simulink model "sim_with_sensors_sim"  (R2023b)
settings: Solver=ode5  StartTime=0.0  StopTime=1000  FixedStep=Auto  RelTol=1e-3
values from neighbouring files (symbols this model uses):
  a = R_E+500*1e3    (= 6871000)    [Sensors.m]    (also in sim_with_sensors.m = 6851.22197053; simulation_with_sensors.m = 26584)
  A0 = eye(3)    [sim_with_sensors.m]
  e = 0    [Sensors.m]    (also in sim_with_sensors.m = 0.00183012221618; simulation_with_sensors.m = 0.00023103)
  H0 = sqrt(g01^2+g11^2+h11^2)*1e-9    [sim_with_sensors.m]    (also in simulation_with_sensors.m)
  I = diag([I1 I2 I3])*1e-9    [sim_with_sensors.m]    (also in simulation_with_sensors.m = diag([100.09 25.1 91.6]))
  Iinv = I\eye(3)    [sim_with_sensors.m]
  incl = deg2rad(11.5)    [sim_with_sensors.m]    (also in simulation_with_sensors.m)
  jb = [0.01; 0.05; 0.01]    [sim_with_sensors.m]
  k_gain = (4*pi/T) * (1 + sin(chsi)) * I1 *1e-9    [sim_with_sensors.m]
  mu = astroConstants(13)    [sim_with_sensors.m]
  n = n+1    (= 1)    [Sensors.m]    (also in sim_with_sensors.m = sqrt(mu/a^3); simulation_with_sensors.m = sqrt(astroConstants(13) / a^3))
  omega0 = [0.01; 0.01; 0.01]*6    [sim_with_sensors.m]
  omegaE = deg2rad(15)/3600    [sim_with_sensors.m]    (also in simulation_with_sensors.m)
  R_mat = om_matrix * i_matrix * OM_matrix    [sim_with_sensors.m]
  Rt = astroConstants(23)    [sim_with_sensors.m]
  s0 = zeros(3,1)    [sim_with_sensors.m]    (also in simulation_with_sensors.m = [0; 0; 0])
  theta0 = 3.109851878856139    (= 3.10985187886)    [sim_with_sensors.m]
undefined symbols (not defined in the file or in its folder): phi0, psi0
libraries: matrix_library x11, simulink x7, dspmathops x6, vrlib x3, dspfdesign x1
settings Model: Creator=marcellopareschi  LastModifiedBy=danie

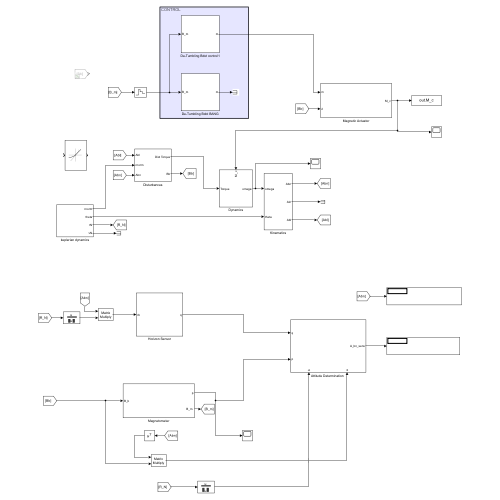
[thumbnail: Simulink's stored preview of the top-level diagram]
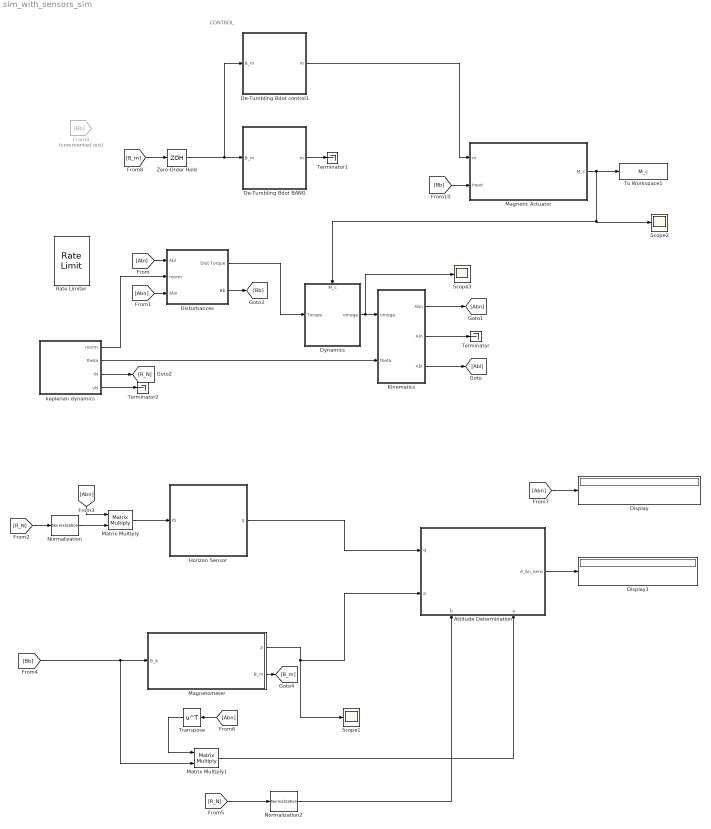
== system sim_with_sensors_sim ==
  note: CONTROL
  "Attitude Determination  " : Subsystem
      settings: PortSchema="{\"entries\":[{\"content\":{\"sides\":[{\"content\":{\"connectorIds\":[\"In1\",\"In2\"]},\"type\":\"ConnectorPlacement.EquallySpacedRectSide\",\"uuid\":\"730966cf-d0d7-44a0-92f0-b5324480e7cc\"},{\"content\":{\"connectorIds\":[\"Out1\"],\"side\":\"RIGHT\"},\"type\":\"ConnectorPlacement.EquallySpacedRectSide\",\"uuid\":\"c83e6b57-46fe-4a45-9824-d3495e15bf6a\"},{\"content\":{\"side\":\"TOP\"},\"type\":\"ConnectorPlacement.EquallySpacedRectSide\",\"uuid\":\"4938c298-c2b3-45b7-bcb0-70b8132dabc6\"},{\"content\":{\"connectorIds\":[\"In3\",\"In4\"],\"side\":\"BOTTOM\"},\"type\":\"ConnectorPlacement.EquallySpacedRectSide\",\"uuid\":\"6d6a244e-80db-423b-a0a5-9a5face48fcb\"}]},\"type\":\"ConnectorPlacement.EquallySpacedConnector\",\"uuid\":\"7eb6767d-3ff0-4577-86c9-ebc5e763f220\"}],\"packageUris\":[\"http://schema.mathworks.com/mf0/Connector/R2020b\"],\"version\":\"1.0\"}"
  De-Tumbling Bdot BANG : Subsystem
  De-Tumbling Bdot control1 : Subsystem
  Display : Display
  Display1 : Display
  Disturbances : Subsystem
  Dynamics : Subsystem
      settings: PortSchema="{\"entries\":[{\"content\":{\"sides\":[{\"content\":{\"connectorIds\":[\"In1\"]},\"type\":\"ConnectorPlacement.EquallySpacedRectSide\",\"uuid\":\"c50eaaef-bc5a-4b30-975a-dad3b72c53e1\"},{\"content\":{\"connectorIds\":[\"Out1\"],\"side\":\"RIGHT\"},\"type\":\"ConnectorPlacement.EquallySpacedRectSide\",\"uuid\":\"08d23e91-5daf-4f03-95f9-71d6696597c3\"},{\"content\":{\"connectorIds\":[\"In2\"],\"side\":\"TOP\"},\"type\":\"ConnectorPlacement.EquallySpacedRectSide\",\"uuid\":\"7ec65280-cc3e-44b1-8843-81c3a216d755\"}]},\"type\":\"ConnectorPlacement.EquallySpacedConnector\",\"uuid\":\"721d018a-ab6c-4a15-8dbf-409a72b03ba1\"}],\"packageUris\":[\"http://schema.mathworks.com/mf0/Connector/R2020b\"],\"version\":\"1.0\"}"
  From9 : From  Commented=on  GotoTag=Bb
  Horizon Sensor : Subsystem
  Kinematics : Subsystem
  Magnetic Actuator : Subsystem
  Magnetometer : Subsystem
  Matrix Multiply : Product  Multiplication=Matrix(*)
  Matrix Multiply1 : Product  Multiplication=Matrix(*)
  Normalization : dspmathops/Normalization  NormType=2-norm  Bias=1e-10  NormOver=Each column  Dimension=1  roundingMode=Floor  overflowMode=off  accumDataTypeStr=Inherit: Same as product output  accumLastDataTypeStr=Inherit: Same as product output  outputDataTypeStr=Inherit: Same as product output  outputMin=[]  outputMax=[]  outputLastDataTypeStr=Inherit: Same as product output
  Normalization2 : dspmathops/Normalization  NormType=2-norm  Bias=1e-10  NormOver=Each column  Dimension=1  roundingMode=Floor  overflowMode=off  accumDataTypeStr=Inherit: Same as product output  accumLastDataTypeStr=Inherit: Same as product output  outputDataTypeStr=Inherit: Same as product output  outputMin=[]  outputMax=[]  outputLastDataTypeStr=Inherit: Same as product output
  Rate Limiter : RateLimiter  SampleTimeMode=inherited
  Scope1 : Scope
  Scope2 : Scope
  Scope3 : Scope
  Terminator : Terminator
  Terminator1 : Terminator
  Terminator2 : Terminator
  To Workspace1 : ToWorkspace  VariableName=M_c  SampleTime=-1
  Transpose : Math  Operator=transpose
  Zero-Order Hold : ZeroOrderHold  SampleTime=1/30
  keplerian dynamics : Subsystem
  wires:
  Dynamics/1(omega) -> Scope3/1, Kinematics/1(omega)
  keplerian dynamics/2(theta) -> Kinematics/2(theta)
  keplerian dynamics/1(rnorm) -> Disturbances/2(rnorm)
  Disturbances/1(Dist Torque) -> Dynamics/1(Torque)
  Kinematics/2(Aln) -> Terminator/1
  Kinematics/3(Abl) -> [Abl]
  [Abl] -> Disturbances/1(Abl)
  Kinematics/1(Abn) -> [Abn]
  [Abn] -> Disturbances/3(Abn)
  keplerian dynamics/4(vN) -> Terminator2/1
  keplerian dynamics/3(rN) -> [R_N]
  [R_N] -> Normalization/1
  Normalization/1 -> Matrix Multiply/2
  [Abn] -> Matrix Multiply/1
  Matrix Multiply/1 -> Horizon Sensor/1(rb)
  Disturbances/2(Bb) -> [Bb]
  [Bb] -> Matrix Multiply1/2, Magnetometer/1(B_b)
  [R_N] -> Normalization2/1
  [Abn] -> Transpose/1
  Transpose/1 -> Matrix Multiply1/1
  Horizon Sensor/1(q) -> "Attitude Determination  "/1(q)
  Magnetometer/1(p) -> Scope1/1, "Attitude Determination  "/2(p)
  Normalization2/1 -> "Attitude Determination  "/3(b)
  Matrix Multiply1/1 -> "Attitude Determination  "/4(a)
  [Abn] -> Display/1
  "Attitude Determination  "/1(A_bn_sens) -> Display1/1
  De-Tumbling Bdot control1/1(m) -> Magnetic Actuator/1(m)
  Magnetometer/2("B_m ") -> [B_m]
  Zero-Order Hold/1 -> De-Tumbling Bdot control1/1(B_m), De-Tumbling Bdot BANG/1(B_m)
  [B_m] -> Zero-Order Hold/1
  [Bb] -> Magnetic Actuator/2(Input)
  De-Tumbling Bdot BANG/1(m) -> Terminator1/1
  Magnetic Actuator/1(M_c) -> Scope2/1, Dynamics/2(M_c), To Workspace1/1

== system sim_with_sensors_sim/Attitude Determination   ==
  q : Inport
  p : Inport  Port=2
  b : Inport  Port=3
  a : Inport  Port=4
  Matrix Multiply : Product  Multiplication=Matrix(*)
  S : Subsystem
  Transpose : Math  Operator=transpose
  V : Subsystem
  A_bn_sens : Outport
  wires:
  q/1 -> S/1(q)
  p/1 -> S/2(p)
  a/1 -> V/2(a)
  b/1 -> V/1(b)
  V/1(V) -> Transpose/1
  S/1(S) -> Matrix Multiply/1
  Transpose/1 -> Matrix Multiply/2
  Matrix Multiply/1 -> A_bn_sens/1

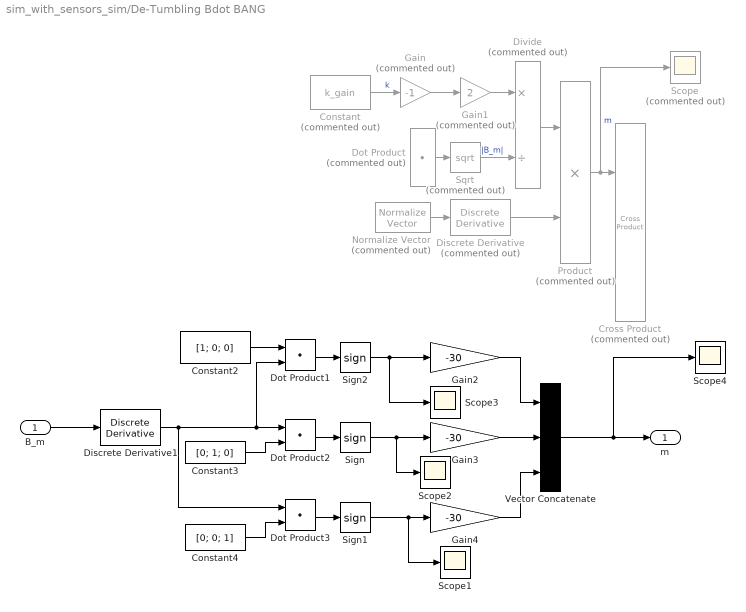
== system sim_with_sensors_sim/De-Tumbling Bdot BANG ==
  B_m : Inport
  Constant : Constant  Commented=on  Value=k_gain
  Constant2 : Constant  Value=[1; 0; 0]  SampleTime=1/30
  Constant3 : Constant  Value=[0; 1; 0]  SampleTime=1/30
  Constant4 : Constant  Value=[0; 0; 1]  SampleTime=1/30
  Cross Product : matrix_library/Cross Product  Commented=on
  Discrete Derivative : simulink/Discrete/Discrete Derivative  Commented=on  gainval=1.0  ICPrevScaledInput=0.0  OutMin=[]  OutMax=[]  OutDataType=fixdt(1, 16)  OutScaling=2^-10  DoSatur=off
  Discrete Derivative1 : simulink/Discrete/Discrete Derivative  gainval=1.0  ICPrevScaledInput=0.0  OutMin=[]  OutMax=[]  OutDataType=fixdt(1, 16)  OutScaling=2^-10  DoSatur=off
  Divide : Product  Commented=on  Inputs=*/
  Dot Product : DotProduct  Commented=on  OutDataTypeStr=Inherit: Inherit via internal rule
  Dot Product1 : DotProduct  OutDataTypeStr=Inherit: Inherit via internal rule
  Dot Product2 : DotProduct  OutDataTypeStr=Inherit: Inherit via internal rule
  Dot Product3 : DotProduct  OutDataTypeStr=Inherit: Inherit via internal rule
  Gain : Gain  Commented=on  Gain=-1
  Gain1 : Gain  Commented=on  Gain=2
  Gain2 : Gain  Gain=-30
  Gain3 : Gain  Gain=-30
  Gain4 : Gain  Gain=-30
  Normalize Vector : vrlib/Utilities/Normalize Vector  Commented=on  maxzero=0
  Product : Product  Commented=on
  Scope : Scope  Commented=on
  Scope{1..4} (4 alike) : Scope
  Sign : Signum
  Sign1 : Signum
  Sign2 : Signum
  Sqrt : Sqrt  Commented=on
  Vector Concatenate : Concatenate  NumInputs=3
  m : Outport
  wires:
  Gain1/1 -> Divide/1
  Normalize Vector/1 -> Discrete Derivative/1
  Sqrt/1 -> Divide/2  "|B_m|"
  Product/1 -> Cross Product/1, Scope/1  "m"
  Discrete Derivative/1 -> Product/2
  Divide/1 -> Product/1
  Gain/1 -> Gain1/1
  Constant/1 -> Gain/1  "k"
  Dot Product/1 -> Sqrt/1
  Discrete Derivative1/1 -> Dot Product3/1, Dot Product2/1, Dot Product1/2
  B_m/1 -> Discrete Derivative1/1
  Constant2/1 -> Dot Product1/1
  Constant3/1 -> Dot Product2/2
  Constant4/1 -> Dot Product3/2
  Dot Product3/1 -> Sign1/1
  Dot Product2/1 -> Sign/1
  Dot Product1/1 -> Sign2/1
  Sign2/1 -> Scope3/1, Gain2/1
  Sign/1 -> Scope2/1, Gain3/1
  Sign1/1 -> Scope1/1, Gain4/1
  Gain3/1 -> Vector Concatenate/2
  Gain4/1 -> Vector Concatenate/3
  Gain2/1 -> Vector Concatenate/1
  Vector Concatenate/1 -> m/1, Scope4/1

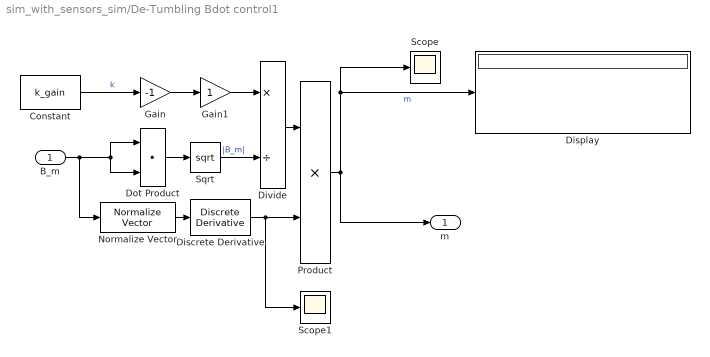
== system sim_with_sensors_sim/De-Tumbling Bdot control1 ==
  B_m : Inport
  Constant : Constant  Value=k_gain
  Discrete Derivative : simulink/Discrete/Discrete Derivative  gainval=1.0  ICPrevScaledInput=0.0  OutMin=[]  OutMax=[]  OutDataType=fixdt(1, 16)  OutScaling=2^-10  DoSatur=off
  Display : Display
  Divide : Product  Inputs=*/
  Dot Product : DotProduct  OutDataTypeStr=Inherit: Inherit via internal rule
  Gain : Gain  Gain=-1
  Gain1 : Gain
  Normalize Vector : vrlib/Utilities/Normalize Vector  maxzero=0
  Product : Product
  Scope : Scope
  Scope1 : Scope
  Sqrt : Sqrt
  m : Outport
  wires:
  Dot Product/1 -> Sqrt/1
  Constant/1 -> Gain/1  "k"
  Gain/1 -> Gain1/1
  Divide/1 -> Product/1
  Discrete Derivative/1 -> Scope1/1, Product/2
  Product/1 -> m/1, Scope/1, Display/1  "m"
  Sqrt/1 -> Divide/2  "|B_m|"
  Gain1/1 -> Divide/1
  Normalize Vector/1 -> Discrete Derivative/1
  B_m/1 -> Normalize Vector/1, Dot Product/2, Dot Product/1

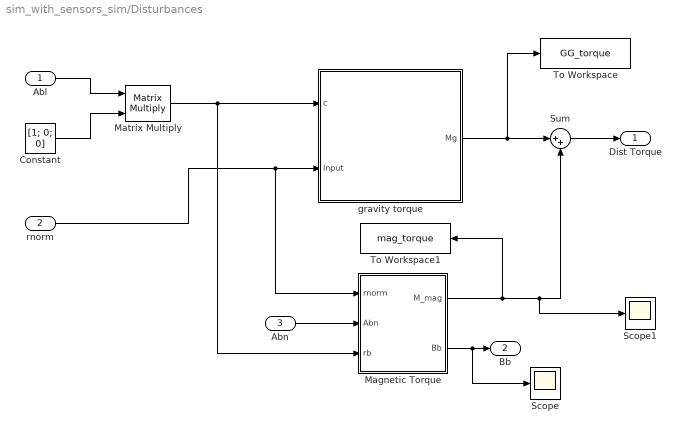
== system sim_with_sensors_sim/Disturbances ==
  Abl : Inport
  rnorm : Inport  Port=2
  Abn : Inport  Port=3
  Constant : Constant  Value=[1; 0; 0]
  "Magnetic Torque " : Subsystem
  Matrix Multiply : Product  Multiplication=Matrix(*)
  Scope : Scope
  Scope1 : Scope
  Sum : Sum  Inputs=|++
  To Workspace : ToWorkspace  VariableName=GG_torque  SampleTime=-1
  To Workspace1 : ToWorkspace  VariableName=mag_torque  SampleTime=-1
  gravity torque : Subsystem
  Dist Torque : Outport
  Bb : Outport  Port=2
  wires:
  Abl/1 -> Matrix Multiply/1
  Constant/1 -> Matrix Multiply/2
  Matrix Multiply/1 -> "Magnetic Torque "/3(rb), gravity torque/1(c)
  rnorm/1 -> "Magnetic Torque "/1(rnorm), gravity torque/2(Input)
  Abn/1 -> "Magnetic Torque "/2(Abn)
  gravity torque/1(Mg) -> To Workspace/1, Sum/1
  "Magnetic Torque "/1(M_mag) -> To Workspace1/1, Scope1/1, Sum/2
  Sum/1 -> Dist Torque/1
  "Magnetic Torque "/2(Bb) -> Scope/1, Bb/1

== system sim_with_sensors_sim/Dynamics ==
  Torque : Inport
  M_c : Inport  Port=2
  Constant : Constant  Value=I
  Constant1 : Constant  Value=Iinv
  Cross Product : matrix_library/Cross Product
  Integrator : Integrator  InitialCondition=omega0
  Product : Product  Multiplication=Matrix(*)
  Product1 : Product  Multiplication=Matrix(*)
  Scope : Scope
  Scope1 : Scope
  Sum : Sum  Inputs=+++
  To Workspace : ToWorkspace  VariableName=omegab  SampleTime=-1
  omega : Outport
  wires:
  Constant/1 -> Product/1
  Product1/1 -> Integrator/1
  Integrator/1 -> omega/1, To Workspace/1, Scope/1, Product/2, Cross Product/2
  Product/1 -> Cross Product/1
  Constant1/1 -> Product1/1
  Cross Product/1 -> Sum/2
  Sum/1 -> Product1/2
  Torque/1 -> Sum/3
  M_c/1 -> Scope1/1, Sum/1

== system sim_with_sensors_sim/Horizon Sensor ==
  rb : Inport
  Cross Product : matrix_library/Cross Product
  Normalization1 : dspmathops/Normalization  NormType=2-norm  Bias=1e-10  NormOver=Each column  Dimension=1  roundingMode=Floor  overflowMode=off  accumDataTypeStr=Inherit: Same as product output  accumLastDataTypeStr=Inherit: Same as product output  outputDataTypeStr=Inherit: Same as product output  outputMin=[]  outputMax=[]  outputLastDataTypeStr=Inherit: Same as product output
  Product : Product
  Sum2 : Sum
  Uniform Random Number : UniformRandomNumber  SampleTime=1/30
  Uniform Random Number1 : UniformRandomNumber  SampleTime=1/30
  Uniform Random Number2 : UniformRandomNumber  SampleTime=1/30
  Uniform Random Number3 : UniformRandomNumber  Minimum=0  Maximum=tan(deg2rad(0.1))  SampleTime=1/30
  Vector Concatenate : Concatenate  NumInputs=3
  Zero-Order Hold : ZeroOrderHold  SampleTime=1/30
  q : Outport
  wires:
  Uniform Random Number/1 -> Vector Concatenate/1
  Product/1 -> Sum2/1
  Uniform Random Number1/1 -> Vector Concatenate/2
  Zero-Order Hold/1 -> Cross Product/2, Sum2/2  "R_B"
  Normalization1/1 -> Product/2
  Vector Concatenate/1 -> Cross Product/1
  Uniform Random Number3/1 -> Product/1
  Cross Product/1 -> Normalization1/1
  Uniform Random Number2/1 -> Vector Concatenate/3
  rb/1 -> Zero-Order Hold/1
  Sum2/1 -> q/1  "q"

== system sim_with_sensors_sim/Kinematics ==
  omega : Inport
  theta : Inport  Port=2
  Product : Product  Multiplication=Matrix(*)
  Subsystem1 : Subsystem
  To Workspace : ToWorkspace  VariableName=angles  SampleTime=-1
  Transpose : Math  Operator=transpose
  compute Aln : Subsystem
  Abn : Outport
  Aln : Outport  Port=2
  Abl : Outport  Port=3
  wires:
  omega/1 -> Subsystem1/1(In1)
  Subsystem1/1(Angles) -> To Workspace/1, Subsystem1/2(Input)
  Subsystem1/2(A) -> Product/1, Abn/1, Subsystem1/3(Input1)
  theta/1 -> compute Aln/1(theta)
  compute Aln/1(A_ln) -> Transpose/1, Aln/1
  Transpose/1 -> Product/2
  Product/1 -> Abl/1

== system sim_with_sensors_sim/Magnetic Actuator ==
  m : Inport
  Input : Inport  Port=2
  Band-Limited White Noise : simulink/Sources/Band-Limited White Noise  Cov=[0.1]  Ts=0.1  seed=[23341]
  Cross Product : matrix_library/Cross Product
  Lowpass Filter : dspfdesign/Lowpass Filter  FilterType=FIR  DesignForMinimumOrder=on  FilterOrder=50  PassbandFrequency=100  StopbandFrequency=120  PassbandRipple=0.1  StopbandAttenuation=80  SampleRateMode=Specify on dialog  SampleRate=44100  SimulateUsing=Interpreted execution  roundingMode=Floor  coeffsDataTypeStr=fixdt(1,16)
  Rate Limiter1 : RateLimiter  RisingSlewLimit=10  FallingSlewLimit=-10  SampleTimeMode=inherited
  Saturation : Saturate  UpperLimit=100  LowerLimit=-100
  Scope1 : Scope
  Sum1 : Sum  Inputs=++|
  M_c : Outport
  wires:
  Input/1 -> Cross Product/2  "B_body"
  Cross Product/1 -> M_c/1
  Rate Limiter1/1 -> Saturation/1
  Band-Limited White Noise/1 -> Sum1/1
  m/1 -> Sum1/2
  Sum1/1 -> Rate Limiter1/1
  Saturation/1 -> Lowpass Filter/1
  Lowpass Filter/1 -> Cross Product/1

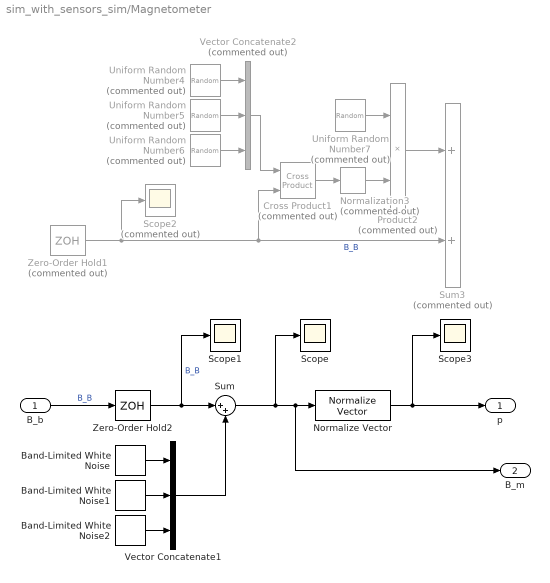
== system sim_with_sensors_sim/Magnetometer ==
  B_b : Inport
  Band-Limited White Noise : simulink/Sources/Band-Limited White Noise  Cov=[1.18^2 *1e-18]  Ts=1/30  seed=[23341]
  Band-Limited White Noise1 : simulink/Sources/Band-Limited White Noise  Cov=[1.18^2 *1e-18]  Ts=1/30  seed=[23341]
  Band-Limited White Noise2 : simulink/Sources/Band-Limited White Noise  Cov=[1.18^2 *1e-18]  Ts=1/30  seed=[23341]
  Cross Product1 : matrix_library/Cross Product  Commented=on
  Normalization3 : dspmathops/Normalization  Commented=on  NormType=2-norm  Bias=1e-10  NormOver=Each column  Dimension=1  roundingMode=Floor  overflowMode=off  accumDataTypeStr=Inherit: Same as product output  accumLastDataTypeStr=Inherit: Same as product output  outputDataTypeStr=Inherit: Same as product output  outputMin=[]  outputMax=[]  outputLastDataTypeStr=Inherit: Same as product output
  Normalize Vector : vrlib/Utilities/Normalize Vector  maxzero=0
  Product2 : Product  Commented=on
  Scope : Scope
  Scope1 : Scope
  Scope2 : Scope  Commented=on
  Scope3 : Scope
  Sum : Sum  Inputs=|++
  Sum3 : Sum  Commented=on
  Uniform Random Number4 : UniformRandomNumber  Commented=on  SampleTime=1/30
  Uniform Random Number5 : UniformRandomNumber  Commented=on  SampleTime=1/30
  Uniform Random Number6 : UniformRandomNumber  Commented=on  SampleTime=1/30
  Uniform Random Number7 : UniformRandomNumber  Commented=on  Minimum=0  Maximum=tan(deg2rad(0.5))  SampleTime=1/30
  Vector Concatenate1 : Concatenate  NumInputs=3
  Vector Concatenate2 : Concatenate  Commented=on  NumInputs=3
  Zero-Order Hold1 : ZeroOrderHold  Commented=on  SampleTime=1/30
  Zero-Order Hold2 : ZeroOrderHold  SampleTime=1/30
  p : Outport
  "B_m " : Outport  Port=2
  wires:
  Zero-Order Hold1/1 -> Cross Product1/2, Sum3/2, Scope2/1  "B_B"
  Product2/1 -> Sum3/1
  Normalization3/1 -> Product2/2
  Uniform Random Number4/1 -> Vector Concatenate2/1
  Uniform Random Number6/1 -> Vector Concatenate2/3
  Vector Concatenate2/1 -> Cross Product1/1
  Cross Product1/1 -> Normalization3/1
  Uniform Random Number5/1 -> Vector Concatenate2/2
  Uniform Random Number7/1 -> Product2/1
  B_b/1 -> Zero-Order Hold2/1  "B_B"
  Zero-Order Hold2/1 -> Scope1/1, Sum/1  "B_B"
  Band-Limited White Noise2/1 -> Vector Concatenate1/3
  Band-Limited White Noise1/1 -> Vector Concatenate1/2
  Band-Limited White Noise/1 -> Vector Concatenate1/1
  Normalize Vector/1 -> Scope3/1, p/1
  Vector Concatenate1/1 -> Sum/2
  Sum/1 -> Scope/1, "B_m "/1, Normalize Vector/1

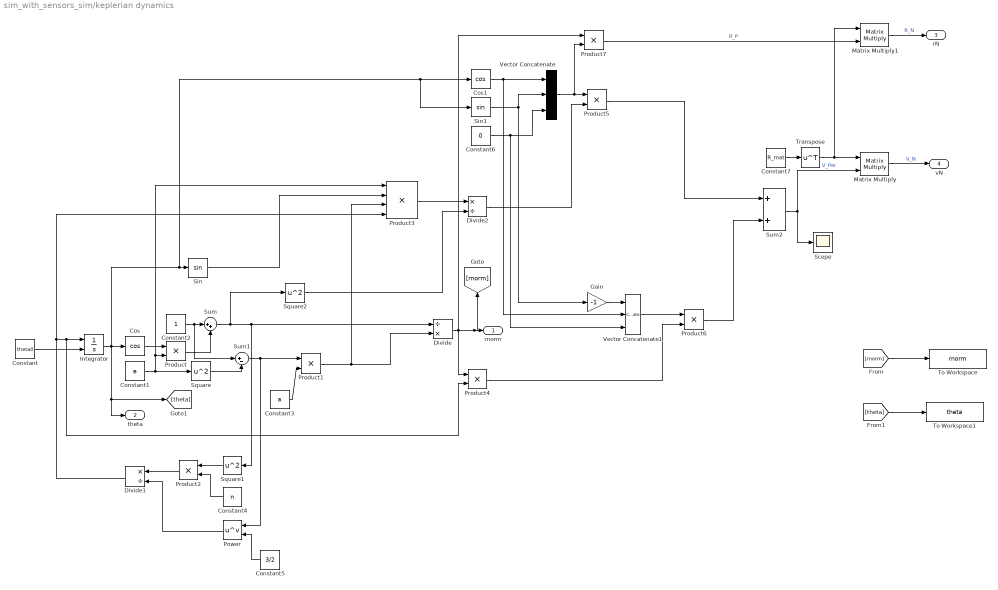
== system sim_with_sensors_sim/keplerian dynamics ==
  Constant : Constant  Value=theta0
  Constant1 : Constant  Value=e
  Constant2 : Constant
  Constant3 : Constant  Value=a
  Constant4 : Constant  Value=n
  Constant5 : Constant  Value=3/2
  Constant6 : Constant  Value=0
  Constant7 : Constant  Value=R_mat
  Cos : Trigonometry  Operator=cos
  Cos1 : Trigonometry  Operator=cos
  Divide : Product  Inputs=/*
  Divide1 : Product  Inputs=*/
  Divide2 : Product  Inputs=*/
  Gain : Gain  Gain=-1
  Integrator : Integrator  InitialConditionSource=external
  Matrix Multiply : Product  Multiplication=Matrix(*)
  Matrix Multiply1 : Product  Multiplication=Matrix(*)
  Power : Math  Operator=pow
  Product{,1..2,4..7} (7 alike) : Product
  Product3 : Product  Inputs=4
  Scope : Scope
  Sin : Trigonometry
  Sin1 : Trigonometry
  Square : Math  Operator=square
  Square1 : Math  Operator=square
  Square2 : Math  Operator=square
  Sum : Sum  Inputs=|++
  Sum1 : Sum  Inputs=|+-
  Sum2 : Sum
  To Workspace : ToWorkspace  VariableName=rnorm  SampleTime=-1
  To Workspace1 : ToWorkspace  VariableName=theta  SampleTime=-1
  Transpose : Math  Operator=transpose
  Vector Concatenate : Concatenate  NumInputs=3
  Vector Concatenate1 : Concatenate  NumInputs=3
  rnorm : Outport
  theta : Outport  Port=2
  rN : Outport  Port=3
  vN : Outport  Port=4
  wires:
  Constant/1 -> Integrator/2
  Integrator/1 -> Sin1/1, Cos1/1, Sin/1, Cos/1, [theta], theta/1
  Cos/1 -> Product/1
  Constant1/1 -> Product3/1, Product/2, Square/1
  Constant2/1 -> Sum1/1, Sum/1
  Product/1 -> Sum/2
  Square/1 -> Sum1/2
  Sum1/1 -> Power/1, Product1/1
  Constant3/1 -> Product1/2
  Product1/1 -> Product3/3, Divide/2
  Sum/1 -> Square2/1, Square1/1, Divide/1
  Square1/1 -> Product2/1
  Constant4/1 -> Product2/2
  Constant5/1 -> Power/2
  Product2/1 -> Divide1/1
  Power/1 -> Divide1/2
  Divide1/1 -> Product3/4, Product4/2, Integrator/1
  Divide/1 -> [rnorm], rnorm/1, Product7/1, Product4/1
  Sin/1 -> Product3/2
  Product3/1 -> Divide2/1
  Square2/1 -> Divide2/2
  Cos1/1 -> Vector Concatenate1/2, Vector Concatenate/1
  Sin1/1 -> Gain/1, Vector Concatenate/2
  Constant6/1 -> Vector Concatenate1/3, Vector Concatenate/3
  Vector Concatenate/1 -> Product7/2, Product5/1
  Divide2/1 -> Product5/2
  Gain/1 -> Vector Concatenate1/1
  Vector Concatenate1/1 -> Product6/1
  Product4/1 -> Product6/2
  Product5/1 -> Sum2/1
  Product6/1 -> Sum2/2
  Constant7/1 -> Transpose/1
  Transpose/1 -> Matrix Multiply1/1, Matrix Multiply/1
  Sum2/1 -> Matrix Multiply/2, Scope/1  "V_Per"
  Product7/1 -> Matrix Multiply1/2  "R_P"
  Matrix Multiply1/1 -> rN/1  "R_N"
  Matrix Multiply/1 -> vN/1  "V_N"
  [rnorm] -> To Workspace/1
  [theta] -> To Workspace1/1

== system sim_with_sensors_sim/Attitude Determination  /S ==
  q : Inport
  p : Inport  Port=2
  Cross Product : matrix_library/Cross Product
  Cross Product1 : matrix_library/Cross Product
  Matrix Concatenate : Concatenate  NumInputs=3  Mode=Multidimensional array  ConcatenateDimension=2
  Normalization : dspmathops/Normalization  NormType=2-norm  Bias=1e-10  NormOver=Each column  Dimension=1  roundingMode=Floor  overflowMode=off  accumDataTypeStr=Inherit: Same as product output  accumLastDataTypeStr=Inherit: Same as product output  outputDataTypeStr=Inherit: Same as product output  outputMin=[]  outputMax=[]  outputLastDataTypeStr=Inherit: Same as product output
  S : Outport
  wires:
  p/1 -> Matrix Concatenate/1, Cross Product/1, Cross Product1/1
  q/1 -> Cross Product/2
  Cross Product/1 -> Normalization/1
  Normalization/1 -> Matrix Concatenate/2, Cross Product1/2
  Matrix Concatenate/1 -> S/1
  Cross Product1/1 -> Matrix Concatenate/3

== system sim_with_sensors_sim/Attitude Determination  /V ==
  b : Inport
  a : Inport  Port=2
  Cross Product : matrix_library/Cross Product
  Cross Product1 : matrix_library/Cross Product
  Matrix Concatenate : Concatenate  NumInputs=3  Mode=Multidimensional array  ConcatenateDimension=2
  Normalization : dspmathops/Normalization  NormType=2-norm  Bias=1e-10  NormOver=Each column  Dimension=1  roundingMode=Floor  overflowMode=off  accumDataTypeStr=Inherit: Same as product output  accumLastDataTypeStr=Inherit: Same as product output  outputDataTypeStr=Inherit: Same as product output  outputMin=[]  outputMax=[]  outputLastDataTypeStr=Inherit: Same as product output
  V : Outport
  wires:
  Cross Product1/1 -> Matrix Concatenate/3
  Matrix Concatenate/1 -> V/1
  Normalization/1 -> Cross Product1/2, Matrix Concatenate/2
  Cross Product/1 -> Normalization/1
  b/1 -> Cross Product/2
  a/1 -> Cross Product1/1, Cross Product/1, Matrix Concatenate/1

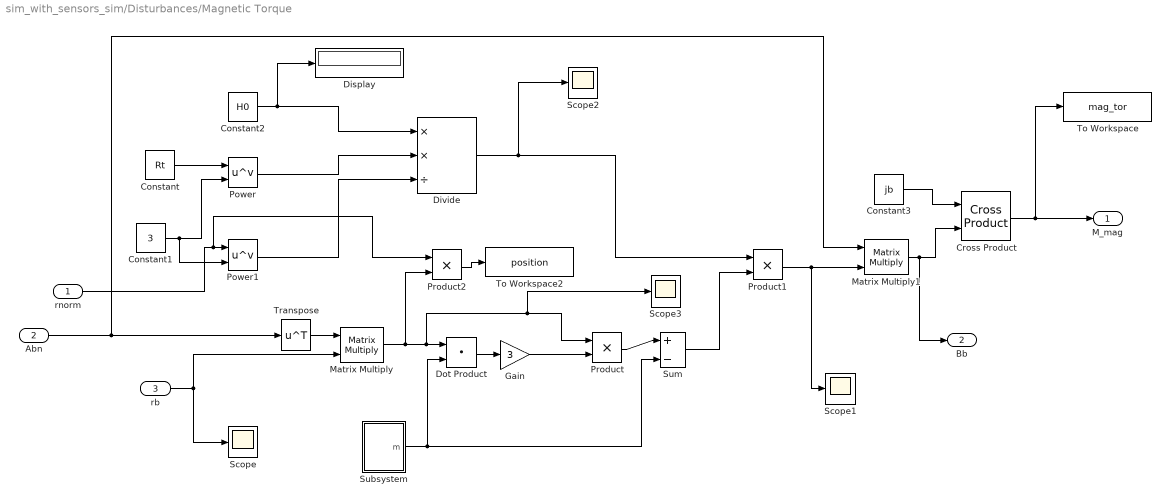
== system sim_with_sensors_sim/Disturbances/Magnetic Torque  ==
  rnorm : Inport
  Abn : Inport  Port=2
  rb : Inport  Port=3
  Constant : Constant  Value=Rt
  Constant1 : Constant  Value=3
  Constant2 : Constant  Value=H0
  Constant3 : Constant  Value=jb
  Cross Product : matrix_library/Cross Product
  Display : Display
  Divide : Product  Inputs=**/
  Dot Product : DotProduct  OutDataTypeStr=Inherit: Inherit via internal rule
  Gain : Gain  Gain=3
  Matrix Multiply : Product  Multiplication=Matrix(*)
  Matrix Multiply1 : Product  Multiplication=Matrix(*)
  Power : Math  Operator=pow
  Power1 : Math  Operator=pow
  Product : Product
  Product1 : Product
  Product2 : Product
  Scope{,1..3} (4 alike) : Scope
  Subsystem : Subsystem
  Sum : Sum  Inputs=|+-
  To Workspace : ToWorkspace  VariableName=mag_tor  SampleTime=-1
  To Workspace2 : ToWorkspace  VariableName=position  SampleTime=-1
  Transpose : Math  Operator=transpose
  M_mag : Outport
  Bb : Outport  Port=2
  wires:
  Abn/1 -> Matrix Multiply1/1, Transpose/1
  Transpose/1 -> Matrix Multiply/1
  rb/1 -> Scope/1, Matrix Multiply/2
  Matrix Multiply/1 -> Product2/2, Scope3/1, Product/1, Dot Product/1
  Subsystem/1(m) -> Sum/2, Dot Product/2
  Dot Product/1 -> Gain/1
  Gain/1 -> Product/2
  Product/1 -> Sum/1
  Constant/1 -> Power/1
  Constant1/1 -> Power1/2, Power/2
  rnorm/1 -> Product2/1, Power1/1
  Constant2/1 -> Display/1, Divide/1
  Power/1 -> Divide/2
  Power1/1 -> Divide/3
  Divide/1 -> Scope2/1, Product1/1
  Sum/1 -> Product1/2
  Product1/1 -> Scope1/1, Matrix Multiply1/2
  Constant3/1 -> Cross Product/1
  Matrix Multiply1/1 -> Bb/1, Cross Product/2
  Cross Product/1 -> To Workspace/1, M_mag/1
  Product2/1 -> To Workspace2/1

== system sim_with_sensors_sim/Disturbances/gravity torque ==
  c : Inport
  Input : Inport  Port=2
  Constant : Constant  Value=mu
  Constant1 : Constant  Value=I
  Constant3 : Constant  Value=3
  Cross Product : matrix_library/Cross Product
  Divide : Product  Inputs=**/
  Gain : Gain  Gain=-1
  Matrix Multiply : Product  Multiplication=Matrix(*)
  Power : Math  Operator=pow
  Product : Product
  Mg : Outport
  wires:
  Constant1/1 -> Matrix Multiply/1
  c/1 -> Matrix Multiply/2, Cross Product/2
  Matrix Multiply/1 -> Cross Product/1
  Constant3/1 -> Power/2, Divide/2
  Power/1 -> Divide/3
  Constant/1 -> Divide/1
  Divide/1 -> Gain/1
  Gain/1 -> Product/2
  Cross Product/1 -> Product/1
  Product/1 -> Mg/1
  Input/1 -> Power/1

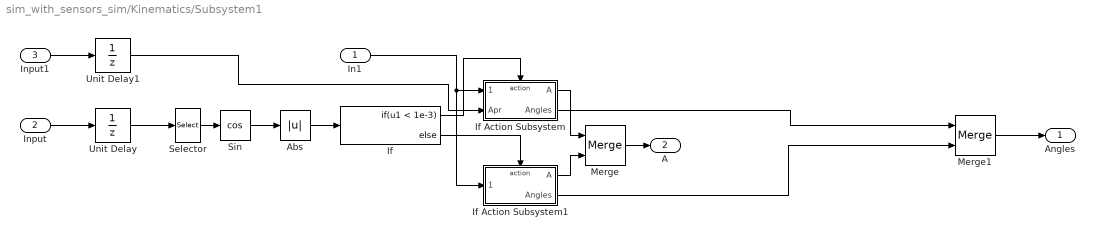
== system sim_with_sensors_sim/Kinematics/Subsystem1 ==
  In1 : Inport
  Input : Inport  Port=2
  Input1 : Inport  Port=3
  Abs : Abs  SaturateOnIntegerOverflow=off
  If : If  IfExpression=u1 < 1e-3
  If Action Subsystem : Subsystem  TreatAsAtomicUnit=on
  If Action Subsystem1 : Subsystem  TreatAsAtomicUnit=on
  Merge : Merge
  Merge1 : Merge
  Selector : Selector  InputPortWidth=3  IndexOptions=Index vector (dialog)  Indices=2  OutputSizes=1
  Sin : Trigonometry  Operator=cos
  Unit Delay : UnitDelay  InitialCondition=s0  SampleTime=-1  HasFrameUpgradeWarning=on
  Unit Delay1 : UnitDelay  InitialCondition=A0  SampleTime=-1  HasFrameUpgradeWarning=on
  Angles : Outport
  A : Outport  Port=2
  wires:
  Input/1 -> Unit Delay/1
  Unit Delay/1 -> Selector/1
  Sin/1 -> Abs/1
  Abs/1 -> If/1
  If/1 -> If Action Subsystem/Action
  If/2 -> If Action Subsystem1/Action
  If Action Subsystem1/1(A) -> Merge/2
  If Action Subsystem/1(A) -> Merge/1
  In1/1 -> If Action Subsystem1/1(omega), If Action Subsystem/1(omega)
  Selector/1 -> Sin/1
  If Action Subsystem1/2(Angles) -> Merge1/2
  If Action Subsystem/2(Angles) -> Merge1/1
  Merge1/1 -> Angles/1
  Merge/1 -> A/1
  Input1/1 -> Unit Delay1/1
  Unit Delay1/1 -> If Action Subsystem/2(Apr)

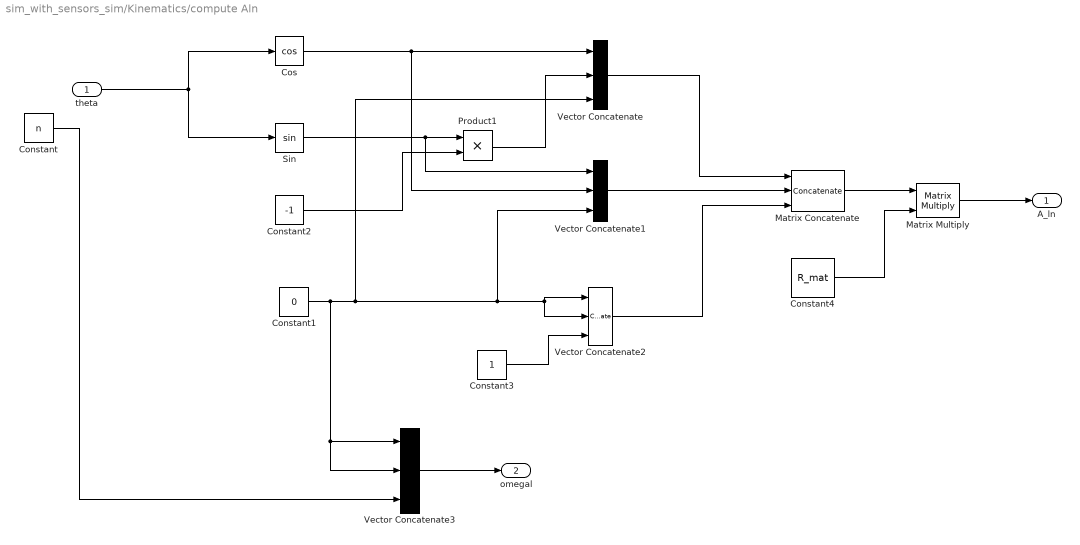
== system sim_with_sensors_sim/Kinematics/compute Aln ==
  theta : Inport
  Constant : Constant  Value=n
  Constant1 : Constant  Value=0
  Constant2 : Constant  Value=-1
  Constant3 : Constant
  Constant4 : Constant  Value=R_mat
  Cos : Trigonometry  Operator=cos
  Matrix Concatenate : Concatenate  NumInputs=3  Mode=Multidimensional array  ConcatenateDimension=2
  Matrix Multiply : Product  Multiplication=Matrix(*)
  Product1 : Product
  Sin : Trigonometry
  Vector Concatenate{,1..3} (4 alike) : Concatenate  NumInputs=3
  A_ln : Outport
  omegal : Outport  Port=2
  wires:
  Constant/1 -> Vector Concatenate3/3
  Cos/1 -> Vector Concatenate1/2, Vector Concatenate/1
  Sin/1 -> Vector Concatenate1/1, Product1/1
  Constant2/1 -> Product1/2
  Product1/1 -> Vector Concatenate/2
  Constant1/1 -> Vector Concatenate3/1, Vector Concatenate3/2, Vector Concatenate/3, Vector Concatenate2/2, Vector Concatenate2/1, Vector Concatenate1/3
  Constant3/1 -> Vector Concatenate2/3
  Vector Concatenate/1 -> Matrix Concatenate/1
  Vector Concatenate1/1 -> Matrix Concatenate/2
  Vector Concatenate2/1 -> Matrix Concatenate/3
  Vector Concatenate3/1 -> omegal/1
  Matrix Concatenate/1 -> Matrix Multiply/1
  Constant4/1 -> Matrix Multiply/2
  Matrix Multiply/1 -> A_ln/1
  theta/1 -> Sin/1, Cos/1

== system sim_with_sensors_sim/Disturbances/Magnetic Torque /Subsystem ==
  Clock : Clock
  Constant : Constant  Value=incl
  Constant1 : Constant  Value=omegaE
  Cos : Trigonometry  Operator=cos
  Cos1 : Trigonometry  Operator=cos
  Product : Product
  Product1 : Product
  Product2 : Product
  Scope : Scope
  Sin : Trigonometry
  Sin1 : Trigonometry
  Vector Concatenate : Concatenate  NumInputs=3
  m : Outport
  wires:
  Constant/1 -> Cos/1, Sin/1
  Clock/1 -> Product/1
  Constant1/1 -> Product/2
  Product/1 -> Sin1/1, Cos1/1
  Cos1/1 -> Product1/1
  Sin/1 -> Product2/2, Product1/2
  Sin1/1 -> Product2/1
  Product1/1 -> Vector Concatenate/1
  Product2/1 -> Vector Concatenate/2
  Cos/1 -> Vector Concatenate/3
  Vector Concatenate/1 -> Scope/1, m/1

== system sim_with_sensors_sim/Kinematics/Subsystem1/If Action Subsystem ==
  omega : Inport
  Apr : Inport  Port=2
  Action Port : ActionPort  ActionPortLabel=if(u1 < 1e-3)
  "Kin 313 " : Subsystem
  conversion 313 312 : Subsystem
  conversion from 312 to 313 : Subsystem
  A : Outport
  Angles : Outport  Port=2
  wires:
  Apr/1 -> conversion from 312 to 313/1(Apr)
  conversion from 312 to 313/1(Angles) -> "Kin 313 "/2(Angles)
  omega/1 -> "Kin 313 "/1(omega)
  "Kin 313 "/1(A) -> conversion 313 312/1(A), A/1
  conversion 313 312/1(Angles) -> Angles/1

== system sim_with_sensors_sim/Kinematics/Subsystem1/If Action Subsystem1 ==
  omega : Inport
  Action Port : ActionPort  ActionPortLabel=else
  Kin 312 : Subsystem
  A : Outport
  Angles : Outport  Port=2
  wires:
  Kin 312/1(A) -> A/1
  omega/1 -> Kin 312/1(omega)
  Kin 312/2(Angles) -> Angles/1

== system sim_with_sensors_sim/Kinematics/Subsystem1/If Action Subsystem/Kin 313  ==
  omega : Inport
  Angles : Inport  Port=2
  Subsystem : Subsystem
  Subsystem1 : Subsystem
  A : Outport
  wires:
  omega/1 -> Subsystem/1(omega)
  Subsystem/1(Phi) -> Subsystem1/1(Phi)
  Subsystem/2(Theta) -> Subsystem1/2(Theta)
  Subsystem/3(Psi) -> Subsystem1/3(Psi)
  Angles/1 -> Subsystem/2(Input)
  Subsystem1/1(A) -> A/1

== system sim_with_sensors_sim/Kinematics/Subsystem1/If Action Subsystem/conversion 313 312 ==
  A : Inport
  Asin : Trigonometry  Operator=asin
  Atan1 : Trigonometry  Operator=atan2
  Atan2 : Trigonometry  Operator=atan2
  Gain : Gain  Gain=-1
  Gain1 : Gain
  Selector : Selector  NumberOfDimensions=2  InputPortWidth=3  IndexOptions=Index vector (dialog),Index vector (dialog)  Indices=1,3  OutputSizes=1,1
  Selector1 : Selector  NumberOfDimensions=2  InputPortWidth=3  IndexOptions=Index vector (dialog),Index vector (dialog)  Indices=3,3  OutputSizes=1,1
  Selector2 : Selector  NumberOfDimensions=2  InputPortWidth=3  IndexOptions=Index vector (dialog),Index vector (dialog)  Indices=2,3  OutputSizes=1,1
  Selector3 : Selector  NumberOfDimensions=2  InputPortWidth=3  IndexOptions=Index vector (dialog),Index vector (dialog)  Indices=2,1  OutputSizes=1,1
  Selector4 : Selector  NumberOfDimensions=2  InputPortWidth=3  IndexOptions=Index vector (dialog),Index vector (dialog)  Indices=2,2  OutputSizes=1,1
  Vector Concatenate : Concatenate  NumInputs=3
  Angles : Outport
  wires:
  Selector/1 -> Gain/1
  Gain/1 -> Atan2/1
  Selector1/1 -> Atan2/2
  A/1 -> Selector1/1, Selector/1, Selector4/1, Selector3/1, Selector2/1
  Selector2/1 -> Asin/1
  Selector3/1 -> Gain1/1
  Gain1/1 -> Atan1/1
  Selector4/1 -> Atan1/2
  Asin/1 -> Vector Concatenate/2
  Atan2/1 -> Vector Concatenate/1
  Atan1/1 -> Vector Concatenate/3
  Vector Concatenate/1 -> Angles/1

== system sim_with_sensors_sim/Kinematics/Subsystem1/If Action Subsystem/conversion from 312 to 313 ==
  Apr : Inport
  Acos : Trigonometry  Operator=acos
  Atan1 : Trigonometry  Operator=atan2
  Atan2 : Trigonometry  Operator=atan2
  Gain : Gain  Gain=-1
  Selector : Selector  NumberOfDimensions=2  InputPortWidth=3  IndexOptions=Index vector (dialog),Index vector (dialog)  Indices=1,3  OutputSizes=1,1
  Selector1 : Selector  NumberOfDimensions=2  InputPortWidth=3  IndexOptions=Index vector (dialog),Index vector (dialog)  Indices=2,3  OutputSizes=1,1
  Selector2 : Selector  NumberOfDimensions=2  InputPortWidth=3  IndexOptions=Index vector (dialog),Index vector (dialog)  Indices=3,3  OutputSizes=1,1
  Selector3 : Selector  NumberOfDimensions=2  InputPortWidth=3  IndexOptions=Index vector (dialog),Index vector (dialog)  Indices=3,2  OutputSizes=1,1
  Selector4 : Selector  NumberOfDimensions=2  InputPortWidth=3  IndexOptions=Index vector (dialog),Index vector (dialog)  Indices=3,1  OutputSizes=1,1
  Vector Concatenate : Concatenate  NumInputs=3
  Angles : Outport
  wires:
  Apr/1 -> Selector/1, Selector1/1, Selector3/1, Selector4/1, Selector2/1
  Selector/1 -> Atan2/1
  Selector1/1 -> Atan2/2
  Selector2/1 -> Acos/1
  Selector4/1 -> Atan1/1
  Acos/1 -> Vector Concatenate/2
  Atan2/1 -> Vector Concatenate/1
  Atan1/1 -> Vector Concatenate/3
  Vector Concatenate/1 -> Angles/1
  Selector3/1 -> Gain/1
  Gain/1 -> Atan1/2

== system sim_with_sensors_sim/Kinematics/Subsystem1/If Action Subsystem1/Kin 312 ==
  omega : Inport
  Euler Angles : Subsystem
  Subsystem : Subsystem
  Vector Concatenate : Concatenate  NumInputs=3
  A : Outport
  Angles : Outport  Port=2
  wires:
  Euler Angles/1(Phi) -> Subsystem/1(phi), Vector Concatenate/3
  Euler Angles/2(Theta) -> Subsystem/2(theta), Vector Concatenate/2
  omega/1 -> Euler Angles/1(omega)
  Euler Angles/3(Psi) -> Subsystem/3(psi), Vector Concatenate/1
  Vector Concatenate/1 -> Angles/1
  Subsystem/1(A) -> A/1

== system sim_with_sensors_sim/Kinematics/Subsystem1/If Action Subsystem/Kin 313 /Subsystem ==
  omega : Inport
  Input : Inport  Port=2
  Demux : Demux  Outputs=3
  phi : Subsystem
  psi : Subsystem
  theta : Subsystem
  Phi : Outport
  Theta : Outport  Port=2
  Psi : Outport  Port=3
  wires:
  phi/1(phi) -> Phi/1
  omega/1 -> psi/1(omega), phi/1(omega), theta/1(omega)
  psi/1(psi) -> theta/2(psi), phi/2(theta), psi/2(Psi), Psi/1
  theta/1(theta) -> Theta/1, psi/3(theta), phi/3(psi)
  Input/1 -> Demux/1
  Demux/1 -> psi/4(Input)
  Demux/2 -> theta/3(Input)
  Demux/3 -> phi/4(Input)

== system sim_with_sensors_sim/Kinematics/Subsystem1/If Action Subsystem/Kin 313 /Subsystem1 ==
  Phi : Inport
  Theta : Inport  Port=2
  Psi : Inport  Port=3
  Product : Product  Inputs=3  Multiplication=Matrix(*)
  R1 : Subsystem
  R3_1 : Subsystem
  R3_2 : Subsystem
  A : Outport
  wires:
  R3_2/1(R3) -> Product/1
  R1/1(R1) -> Product/2
  R3_1/1(R3) -> Product/3
  Phi/1 -> R3_1/1(x)
  Theta/1 -> R1/1(x)
  Psi/1 -> R3_2/1(x)
  Product/1 -> A/1

== system sim_with_sensors_sim/Kinematics/Subsystem1/If Action Subsystem1/Kin 312/Euler Angles ==
  omega : Inport
  Constant : Constant  Value=s0
  Demux : Demux  Outputs=3
  phi : Subsystem
  psi : Subsystem
  th : Subsystem
  Phi : Outport
  Theta : Outport  Port=2
  Psi : Outport  Port=3
  wires:
  th/1(theta) -> Theta/1, psi/2(Th), phi/2(th)
  psi/1(psi) -> phi/3(psi), th/2(psi), psi/3(psi_), Psi/1
  phi/1(phi) -> Phi/1
  omega/1 -> psi/1(omega), phi/1(omega), th/1(omega)
  Demux/3 -> phi/4(In4)
  Demux/2 -> th/3(In3)
  Demux/1 -> psi/4(In4)
  Constant/1 -> Demux/1

== system sim_with_sensors_sim/Kinematics/Subsystem1/If Action Subsystem1/Kin 312/Subsystem ==
  phi : Inport
  theta : Inport  Port=2
  psi : Inport  Port=3
  Product : Product  Inputs=3  Multiplication=Matrix(*)
  R1 : Subsystem
  R2 : Subsystem
  R3 : Subsystem
  A : Outport
  wires:
  R1/1(R1) -> Product/2
  R3/1(R3) -> Product/3
  R2/1(R2) -> Product/1
  phi/1 -> R3/1(x)
  theta/1 -> R1/1(x)
  psi/1 -> R2/1(x)
  Product/1 -> A/1

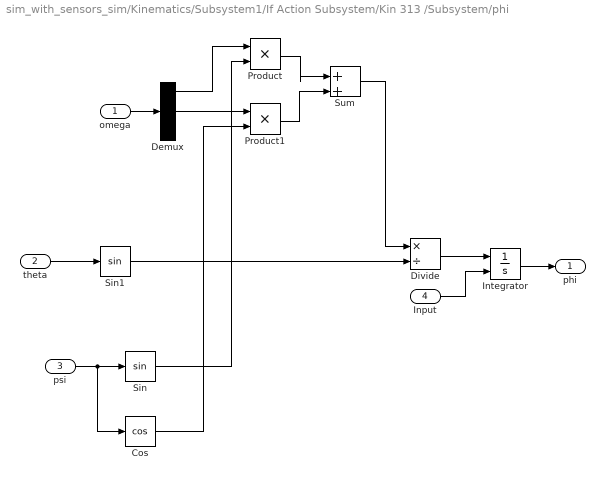
== system sim_with_sensors_sim/Kinematics/Subsystem1/If Action Subsystem/Kin 313 /Subsystem/phi ==
  omega : Inport
  theta : Inport  Port=2
  psi : Inport  Port=3
  Input : Inport  Port=4
  Cos : Trigonometry  Operator=cos
  Demux : Demux  Outputs=3
  Divide : Product  Inputs=*/
  Integrator : Integrator  InitialConditionSource=external  WrappedStateUpperValue=2*pi  WrappedStateLowerValue=0
  Product : Product
  Product1 : Product
  Sin : Trigonometry
  Sin1 : Trigonometry
  Sum : Sum  Inputs=|++
  phi : Outport
  wires:
  omega/1 -> Demux/1
  Demux/1 -> Product/1
  psi/1 -> Cos/1, Sin/1
  Sin/1 -> Product/2
  Demux/2 -> Product1/1
  Cos/1 -> Product1/2
  Product/1 -> Sum/1
  Product1/1 -> Sum/2
  theta/1 -> Sin1/1
  Sum/1 -> Divide/1
  Sin1/1 -> Divide/2
  Divide/1 -> Integrator/1
  Integrator/1 -> phi/1
  Input/1 -> Integrator/2

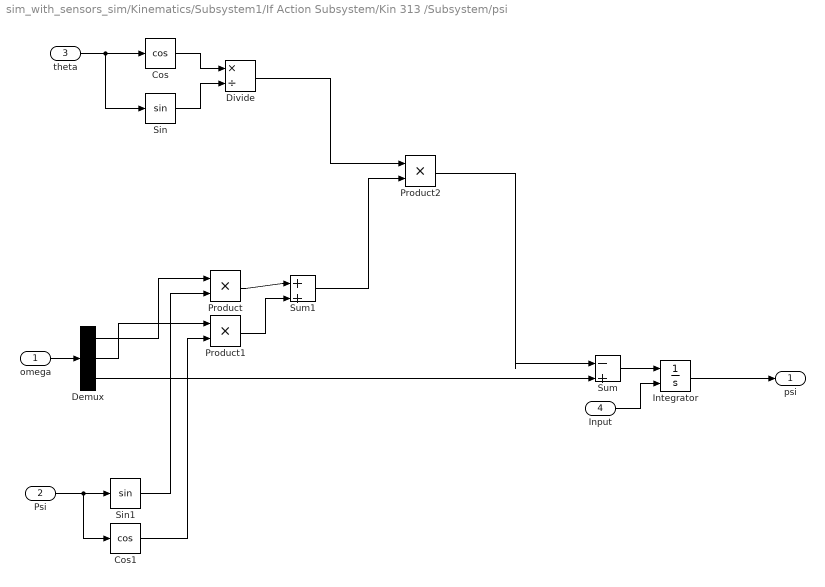
== system sim_with_sensors_sim/Kinematics/Subsystem1/If Action Subsystem/Kin 313 /Subsystem/psi ==
  omega : Inport
  Psi : Inport  Port=2
  theta : Inport  Port=3
  Input : Inport  Port=4
  Cos : Trigonometry  Operator=cos
  Cos1 : Trigonometry  Operator=cos
  Demux : Demux  Outputs=3
  Divide : Product  Inputs=*/
  Integrator : Integrator  InitialConditionSource=external  WrappedStateUpperValue=2*pi  WrappedStateLowerValue=0
  Product : Product
  Product1 : Product
  Product2 : Product
  Sin : Trigonometry
  Sin1 : Trigonometry
  Sum : Sum  Inputs=|-+
  Sum1 : Sum  Inputs=|++
  psi : Outport
  wires:
  omega/1 -> Demux/1
  theta/1 -> Sin/1, Cos/1
  Cos/1 -> Divide/1
  Sin/1 -> Divide/2
  Psi/1 -> Sin1/1, Cos1/1
  Demux/1 -> Product/1
  Sin1/1 -> Product/2
  Demux/2 -> Product1/1
  Cos1/1 -> Product1/2
  Product/1 -> Sum1/1
  Product1/1 -> Sum1/2
  Divide/1 -> Product2/1
  Sum1/1 -> Product2/2
  Demux/3 -> Sum/2
  Product2/1 -> Sum/1
  Sum/1 -> Integrator/1
  Integrator/1 -> psi/1
  Input/1 -> Integrator/2

== system sim_with_sensors_sim/Kinematics/Subsystem1/If Action Subsystem/Kin 313 /Subsystem/theta ==
  omega : Inport
  psi : Inport  Port=2
  Input : Inport  Port=3
  Cos : Trigonometry  Operator=cos
  Demux : Demux  Outputs=3
  Integrator : Integrator  InitialConditionSource=external  WrappedStateUpperValue=2*pi  WrappedStateLowerValue=0
  Product : Product
  Product1 : Product
  Sin : Trigonometry
  Sum : Sum  Inputs=|++
  theta : Outport
  wires:
  omega/1 -> Demux/1
  psi/1 -> Cos/1, Sin/1
  Demux/1 -> Product/1
  Sin/1 -> Product/2
  Demux/2 -> Product1/1
  Cos/1 -> Product1/2
  Product/1 -> Sum/1
  Product1/1 -> Sum/2
  Sum/1 -> Integrator/1
  Integrator/1 -> theta/1
  Input/1 -> Integrator/2

== system sim_with_sensors_sim/Kinematics/Subsystem1/If Action Subsystem/Kin 313 /Subsystem1/R1 ==
  x : Inport
  Constant : Constant  Value=[1; 0; 0]
  Constant1 : Constant  Value=0
  Cos : Trigonometry  Operator=cos
  Gain : Gain  Gain=-1
  Matrix Concatenate : Concatenate  NumInputs=3  Mode=Multidimensional array  ConcatenateDimension=2
  Sin : Trigonometry
  Vector Concatenate : Concatenate  NumInputs=3
  Vector Concatenate1 : Concatenate  NumInputs=3
  R1 : Outport
  wires:
  Sin/1 -> Gain/1, Vector Concatenate/2
  Gain/1 -> Vector Concatenate1/3
  Cos/1 -> Vector Concatenate1/2, Vector Concatenate/3
  Constant1/1 -> Vector Concatenate1/1, Vector Concatenate/1
  Vector Concatenate/1 -> Matrix Concatenate/3
  Constant/1 -> Matrix Concatenate/1
  Vector Concatenate1/1 -> Matrix Concatenate/2
  x/1 -> Sin/1, Cos/1
  Matrix Concatenate/1 -> R1/1

== system sim_with_sensors_sim/Kinematics/Subsystem1/If Action Subsystem/Kin 313 /Subsystem1/R3_1 ==
  x : Inport
  Constant : Constant  Value=[0; 0; 1]
  Constant1 : Constant  Value=0
  Cos : Trigonometry  Operator=cos
  Gain : Gain  Gain=-1
  Matrix Concatenate : Concatenate  NumInputs=3  Mode=Multidimensional array  ConcatenateDimension=2
  Sin : Trigonometry
  Vector Concatenate : Concatenate  NumInputs=3
  Vector Concatenate1 : Concatenate  NumInputs=3
  R3 : Outport
  wires:
  Matrix Concatenate/1 -> R3/1
  Constant1/1 -> Vector Concatenate1/3, Vector Concatenate/3
  x/1 -> Cos/1, Sin/1
  Vector Concatenate1/1 -> Matrix Concatenate/2
  Gain/1 -> Vector Concatenate/2
  Constant/1 -> Matrix Concatenate/3
  Cos/1 -> Vector Concatenate/1, Vector Concatenate1/2
  Sin/1 -> Gain/1, Vector Concatenate1/1
  Vector Concatenate/1 -> Matrix Concatenate/1

== system sim_with_sensors_sim/Kinematics/Subsystem1/If Action Subsystem/Kin 313 /Subsystem1/R3_2 ==
  x : Inport
  Constant : Constant  Value=[0; 0; 1]
  Constant1 : Constant  Value=0
  Cos : Trigonometry  Operator=cos
  Gain : Gain  Gain=-1
  Matrix Concatenate : Concatenate  NumInputs=3  Mode=Multidimensional array  ConcatenateDimension=2
  Sin : Trigonometry
  Vector Concatenate : Concatenate  NumInputs=3
  Vector Concatenate1 : Concatenate  NumInputs=3
  R3 : Outport
  wires:
  Vector Concatenate/1 -> Matrix Concatenate/1
  Sin/1 -> Vector Concatenate1/1, Gain/1
  Cos/1 -> Vector Concatenate1/2, Vector Concatenate/1
  Constant/1 -> Matrix Concatenate/3
  Gain/1 -> Vector Concatenate/2
  Vector Concatenate1/1 -> Matrix Concatenate/2
  x/1 -> Sin/1, Cos/1
  Constant1/1 -> Vector Concatenate/3, Vector Concatenate1/3
  Matrix Concatenate/1 -> R3/1

== system sim_with_sensors_sim/Kinematics/Subsystem1/If Action Subsystem1/Kin 312/Euler Angles/phi ==
  omega : Inport
  th : Inport  Port=2
  psi : Inport  Port=3
  In4 : Inport  Port=4
  Cos : Trigonometry  Operator=cos
  Cos1 : Trigonometry  Operator=cos
  Demux : Demux  Outputs=3
  Divide : Product  Inputs=*/
  Integrator : Integrator  InitialConditionSource=external  InitialCondition=phi0  WrappedStateUpperValue=2*pi  WrappedStateLowerValue=0
  Product : Product
  Product1 : Product
  Sin : Trigonometry
  Sum : Sum  Inputs=|-+
  phi : Outport
  wires:
  omega/1 -> Demux/1
  psi/1 -> Cos/1, Sin/1
  Demux/1 -> Product/1
  Sin/1 -> Product/2
  Demux/3 -> Product1/1
  Cos/1 -> Product1/2
  Product/1 -> Sum/1
  Product1/1 -> Sum/2
  th/1 -> Cos1/1
  Sum/1 -> Divide/1
  Cos1/1 -> Divide/2
  Divide/1 -> Integrator/1
  Integrator/1 -> phi/1
  In4/1 -> Integrator/2

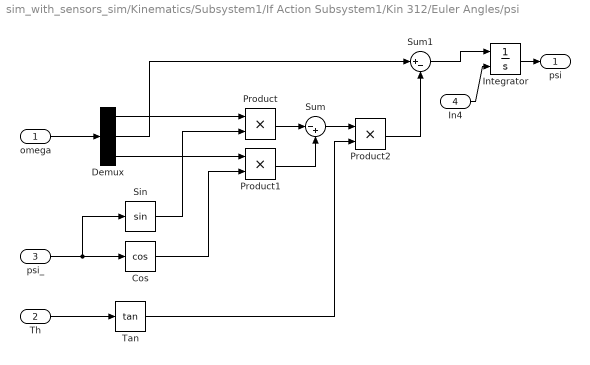
== system sim_with_sensors_sim/Kinematics/Subsystem1/If Action Subsystem1/Kin 312/Euler Angles/psi ==
  omega : Inport
  Th : Inport  Port=2
  psi_ : Inport  Port=3
  In4 : Inport  Port=4
  Cos : Trigonometry  Operator=cos
  Demux : Demux  Outputs=3
  Integrator : Integrator  InitialConditionSource=external  InitialCondition=psi0  WrappedStateUpperValue=2*pi  WrappedStateLowerValue=0
  Product : Product
  Product1 : Product
  Product2 : Product
  Sin : Trigonometry
  Sum : Sum  Inputs=|-+
  Sum1 : Sum  Inputs=|+-
  Tan : Trigonometry  Operator=tan
  psi : Outport
  wires:
  omega/1 -> Demux/1
  psi_/1 -> Sin/1, Cos/1
  Demux/1 -> Product/1
  Sin/1 -> Product/2
  Demux/3 -> Product1/1
  Cos/1 -> Product1/2
  Th/1 -> Tan/1
  Product/1 -> Sum/1
  Product1/1 -> Sum/2
  Sum/1 -> Product2/1
  Tan/1 -> Product2/2
  Product2/1 -> Sum1/2
  Demux/2 -> Sum1/1
  Sum1/1 -> Integrator/1
  Integrator/1 -> psi/1
  In4/1 -> Integrator/2

== system sim_with_sensors_sim/Kinematics/Subsystem1/If Action Subsystem1/Kin 312/Euler Angles/th ==
  omega : Inport
  psi : Inport  Port=2
  In3 : Inport  Port=3
  Cos : Trigonometry  Operator=cos
  Demux : Demux  Outputs=3
  Integrator : Integrator  InitialConditionSource=external  InitialCondition=theta0  WrappedStateUpperValue=2*pi  WrappedStateLowerValue=0
  Product : Product
  Product1 : Product
  Sin : Trigonometry
  Sum : Sum  Inputs=|++
  theta : Outport
  wires:
  omega/1 -> Demux/1
  psi/1 -> Sin/1, Cos/1
  Demux/1 -> Product/1
  Cos/1 -> Product/2
  Demux/3 -> Product1/1
  Sin/1 -> Product1/2
  Product/1 -> Sum/1
  Product1/1 -> Sum/2
  Sum/1 -> Integrator/1
  Integrator/1 -> theta/1
  In3/1 -> Integrator/2

== system sim_with_sensors_sim/Kinematics/Subsystem1/If Action Subsystem1/Kin 312/Subsystem/R1 ==
  x : Inport
  Constant : Constant  Value=[1; 0; 0]
  Constant1 : Constant  Value=0
  Cos : Trigonometry  Operator=cos
  Gain : Gain  Gain=-1
  Matrix Concatenate : Concatenate  NumInputs=3  Mode=Multidimensional array  ConcatenateDimension=2
  Sin : Trigonometry
  Vector Concatenate : Concatenate  NumInputs=3
  Vector Concatenate1 : Concatenate  NumInputs=3
  R1 : Outport
  wires:
  Matrix Concatenate/1 -> R1/1
  x/1 -> Cos/1, Sin/1
  Vector Concatenate1/1 -> Matrix Concatenate/2
  Constant/1 -> Matrix Concatenate/1
  Vector Concatenate/1 -> Matrix Concatenate/3
  Constant1/1 -> Vector Concatenate/1, Vector Concatenate1/1
  Cos/1 -> Vector Concatenate/3, Vector Concatenate1/2
  Gain/1 -> Vector Concatenate1/3
  Sin/1 -> Vector Concatenate/2, Gain/1

== system sim_with_sensors_sim/Kinematics/Subsystem1/If Action Subsystem1/Kin 312/Subsystem/R2 ==
  x : Inport
  Constant : Constant  Value=[0; 1; 0]
  Constant1 : Constant  Value=0
  Cos : Trigonometry  Operator=cos
  Gain : Gain  Gain=-1
  Matrix Concatenate : Concatenate  NumInputs=3  Mode=Multidimensional array  ConcatenateDimension=2
  Sin : Trigonometry
  Vector Concatenate : Concatenate  NumInputs=3
  Vector Concatenate1 : Concatenate  NumInputs=3
  R2 : Outport
  wires:
  Vector Concatenate/1 -> Matrix Concatenate/1
  x/1 -> Sin/1, Cos/1
  Matrix Concatenate/1 -> R2/1
  Constant/1 -> Matrix Concatenate/2
  Vector Concatenate1/1 -> Matrix Concatenate/3
  Constant1/1 -> Vector Concatenate/2, Vector Concatenate1/2
  Cos/1 -> Vector Concatenate1/3, Vector Concatenate/1
  Sin/1 -> Gain/1, Vector Concatenate/3
  Gain/1 -> Vector Concatenate1/1

== system sim_with_sensors_sim/Kinematics/Subsystem1/If Action Subsystem1/Kin 312/Subsystem/R3 ==
  x : Inport
  Constant : Constant  Value=[0; 0; 1]
  Constant1 : Constant  Value=0
  Cos : Trigonometry  Operator=cos
  Gain : Gain  Gain=-1
  Matrix Concatenate : Concatenate  NumInputs=3  Mode=Multidimensional array  ConcatenateDimension=2
  Sin : Trigonometry
  Vector Concatenate : Concatenate  NumInputs=3
  Vector Concatenate1 : Concatenate  NumInputs=3
  R3 : Outport
  wires:
  Vector Concatenate/1 -> Matrix Concatenate/1
  Sin/1 -> Vector Concatenate1/1, Gain/1
  Cos/1 -> Vector Concatenate1/2, Vector Concatenate/1
  Constant/1 -> Matrix Concatenate/3
  Gain/1 -> Vector Concatenate/2
  Vector Concatenate1/1 -> Matrix Concatenate/2
  x/1 -> Sin/1, Cos/1
  Constant1/1 -> Vector Concatenate/3, Vector Concatenate1/3
  Matrix Concatenate/1 -> R3/1
